simulink model "system3_"  (R2018b)
settings: Solver=VariableStepAuto  StartTime=0.0  StopTime=30  RelTol=1e-3
libraries: cstblocks x2
settings Model: Creator=Abraham Pérez  LastModifiedBy=Abraham Pérez

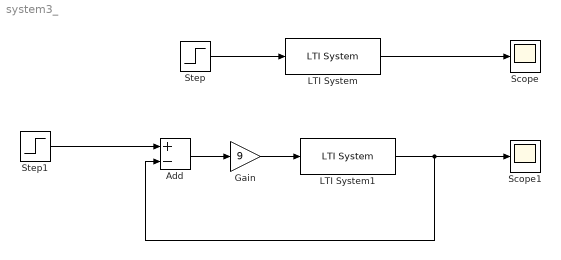
== system system3_ ==
  Add : Sum  Inputs=+-
  Gain : Gain  Gain=9
  LTI System : cstblocks/LTI System  sys=G3  IC=[]
  LTI System1 : cstblocks/LTI System  sys=G3  IC=[]
  Scope : Scope
  Scope1 : Scope
  Step : Step  Time=0  Before=8.5  After=8.5  SampleTime=0
  Step1 : Step  Time=0  Before=17  After=17  SampleTime=0
  wires:
  Step/1 -> LTI System/1
  Gain/1 -> LTI System1/1
  Add/1 -> Gain/1
  Step1/1 -> Add/1
  LTI System/1 -> Scope/1
  LTI System1/1 -> Scope1/1, Add/2
